simulink library "libMatUdp"  (R2015a)
settings: Solver=ode45  StartTime=0.0  StopTime=10.0  RelTol=1e-3
undefined symbols (not defined in the file): BusSerialize, gcbh, mxpcrtudprx
libraries: xpcnetworkbufferlib x5, xpciplib x4
settings Model: Creator=djoshea  LastModifiedBy=djoshea

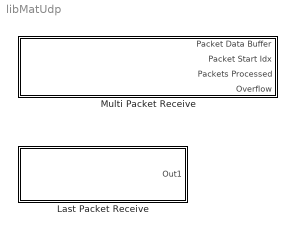
== system libMatUdp ==
  "Last Packet Receive " : Subsystem  InitFcn=mxpcrtudprx(1, get_param(gcbh, 'ID'));  mask(rtudpreceive){maskID=1, sourceIP='0.0.0.0', Receive2=25000, Receive3=1500, Receive4=-1, udpID=0, ID=1}
      mask prompts: maskID "Device ID"; sourceIP "Source IP Address:"; Receive2 "Local (destination) port:"; Receive3 "Output port width:"; Receive4 "Sample time:"; udpID "Internal UDP ID:"; ID "Device ID:"
      mask help:
      | Receive data over UDP network.
      |
      | This block receives data on the specified local (destination) port. To receive all data sent to this port, set 'Source IP Address' to 0.0.0.0. To receive data sent to this port from a specific remote source, enter that IP address.
      mask init:
      | set(gcbh, 'ID', num2str(maskID));
      | set(gcbh, 'Receive1', sourceIP);
      mask TypeOptions Receive2: Receive2
      mask TypeOptions Receive3: Receive3
      mask TypeOptions Receive4: Receive4
      mask TypeOptions udpID: udpID
      mask TypeOptions ID: ID
      mask Display:
      | try
      |     disp(sprintf('UDP Receive\nDevice ID: %d\n%s to port %d', maskID, sourceIP, Receive2));
      | catch
      |     disp('UDP Receive');
      | end
      | port_label('output', 1, 'Data');
  "Multi Packet Receive " : Subsystem  InitFcn=mxpcrtudprx(1, get_param(gcbh, 'ID'));  mask(rtudpreceive){ID=1, sourceIP=0.0.0.0, recvPort=25000, PacketDataBufferMaxSize=15000, PacketChainSize=20, PacketBufferSize=0, Receive4=0.001, udpID=0}
      mask prompts: ID "Device ID:"; sourceIP "Source IP Address:"; recvPort "Local (destination) port:"; PacketDataBufferMaxSize "Packet Data Buffer Max Size:"; PacketChainSize "Packet Chain Size"; PacketBufferSize "Packet Buffer Size"; Receive4 "Sample time:"; udpID "Internal UDP ID:"
      mask help:
      | Receive data over UDP network on a dedicated network interface.
      |
      | This block receives data on the specified local (destination) port. To receive all data sent to this port, set 'Source IP Address' to 0.0.0.0. To receive data sent to this port from a specific remote source, enter the IP address of that source.
      mask init:
      | udpID = ID -1;
      mask Help: eval('xpcdoc(''RT_UDP_RECEIVE'')');
      mask TypeOptions ID: 1 | 2 | 3 | 4 | 5 | 6 | 7 | 8
      mask Display:
      | try
      |     disp(sprintf('Multi-UDP Receive\nDevice Id: %d\n%s to port %d', ...
      |         ID, BusSerialize.ipStringFromAddress(sourceIP), recvPort));
      | catch
      |     disp('Multi-UDP Receive');
      | end
      | port_label('output', 1, 'Data');
      | port_label('output', 2, 'Start Idx');
      | port_label('output', 3, 'Packet Count');
      | port_label('output', 4, 'Overflow');

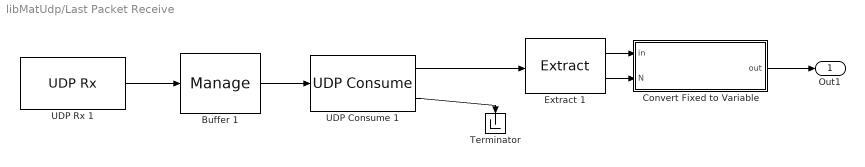
== system libMatUdp/Last Packet Receive  ==
  Buffer 1 : xpcnetworkbufferlib/Manage   ChainSize=-1  BufferSize=0  Threshold=0
  Convert Fixed to Variable : MATLAB Function  TreatAsAtomicUnit=on  mask(Converts Variable-size to fixed-size array){bufferSize=1500}
      mask prompts: bufferSize "Buffer Size"
      mask help: Specify maximum input size.
  Extract 1 : xpcnetworkbufferlib/Extract   PacketSize=Receive3
  Terminator : Terminator
  UDP Consume 1 : xpciplib/UDP Consume   Group=udpID  VectorSize=0  SampleTime=Receive4
  UDP Rx 1 : xpciplib/UDP Rx   Priority=5  Group=udpID  sip=Any  SourceAddress=Receive1  lup=Specify  LocalPort=Receive2  SampleTime=Receive4
  Out1 : Outport  OutDataTypeStr=uint8
  wires:
  Extract 1/1 -> Convert Fixed to Variable/1(in)
  Buffer 1/1 -> UDP Consume 1/1
  UDP Rx 1/1 -> Buffer 1/1
  UDP Consume 1/1 -> Extract 1/1
  UDP Consume 1/2 -> Terminator/1
  Extract 1/2 -> Convert Fixed to Variable/2(N)
  Convert Fixed to Variable/1(out) -> Out1/1

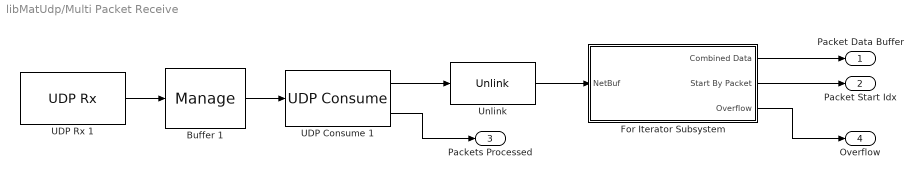
== system libMatUdp/Multi Packet Receive  ==
  Buffer 1 : xpcnetworkbufferlib/Manage   ChainSize=PacketChainSize  BufferSize=PacketBufferSize  Threshold=0
  For Iterator Subsystem : Subsystem  TreatAsAtomicUnit=on
  UDP Consume 1 : xpciplib/UDP Consume   Group=udpID  VectorSize=0  SampleTime=Receive4
  UDP Rx 1 : xpciplib/UDP Rx   Priority=5  Group=udpID  sip=Any  SourceAddress=BusSerialize.ipAddressFromString(sourceIP)  lup=Specify  LocalPort=recvPort  SampleTime=Receive4
  "Unlink " : xpcnetworkbufferlib/Unlink   VectorLength=-1
  Packet Data Buffer : Outport
  Packet Start Idx : Outport  Port=2
  Packets Processed : Outport  Port=3
  Overflow : Outport  Port=4
  wires:
  For Iterator Subsystem/3(Overflow) -> Overflow/1
  For Iterator Subsystem/2(Start By Packet) -> Packet Start Idx/1
  For Iterator Subsystem/1(Combined Data) -> Packet Data Buffer/1
  "Unlink "/1 -> For Iterator Subsystem/1(NetBuf)
  Buffer 1/1 -> UDP Consume 1/1
  UDP Rx 1/1 -> Buffer 1/1
  UDP Consume 1/1 -> "Unlink "/1
  UDP Consume 1/2 -> Packets Processed/1

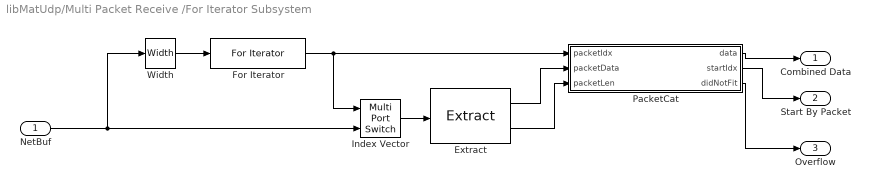
== system libMatUdp/Multi Packet Receive /For Iterator Subsystem ==
  NetBuf : Inport
  "Extract " : xpcnetworkbufferlib/Extract   PacketSize=-1
  For Iterator : ForIterator  ResetStates=reset  IterationSource=external
  Index Vector : MultiPortSwitch  DataPortOrder=Zero-based contiguous  Inputs=1  zeroidx=on
  PacketCat : MATLAB Function  TreatAsAtomicUnit=on
  Width : Width
  Combined Data : Outport
  Start By Packet : Outport  Port=2
  Overflow : Outport  Port=3  OutDataTypeStr=uint8
  wires:
  PacketCat/3(didNotFit) -> Overflow/1
  PacketCat/2(startIdx) -> Start By Packet/1
  PacketCat/1(data) -> Combined Data/1
  "Extract "/2 -> PacketCat/3(packetLen)
  "Extract "/1 -> PacketCat/2(packetData)
  Index Vector/1 -> "Extract "/1
  For Iterator/1 -> PacketCat/1(packetIdx), Index Vector/1
  Width/1 -> For Iterator/1
  NetBuf/1 -> Width/1, Index Vector/2

== matlab function libMatUdp/Multi Packet Receive /For Iterator Subsystem/PacketCat ==
  data: packetIdx input; data output uint8 size=PacketDataBufferMaxSize; packetData input uint8; packetLen input size=1; startIdx output size=PacketChainSize; PacketDataBufferMaxSize parameter size=1; PacketChainSize parameter size=1; didNotFit output uint8 size=1
function [data, startIdx, didNotFit] = packetCat(packetIdx, packetData, packetLen, PacketDataBufferMaxSize, PacketChainSize)
%#codegen

persistent pData;
persistent pDataLen;
persistent pStartIdx;
persistent pStartIdxLen;
persistent pDidNotFit;

if packetIdx == 1 || isempty(pData) || isempty(pDataLen) || isempty(pStartIdx) || isempty(pStartIdxLen) || isempty(pDidNotFit)
    pData = coder.nullcopy(zeros(PacketDataBufferMaxSize, 1, 'uint8'));
    pDataLen = uint32(0);
    pStartIdx = coder.nullcopy(zeros(PacketChainSize, 1, 'uint32'));
    pStartIdxLen = uint16(0);
    pDidNotFit = uint8(0);
end

% check whether there is room for this packet
canFitBytes = numel(pData) - pDataLen >= packetLen;
canFitPacket = numel(pStartIdx) - pStartIdxLen > 0;
if canFitBytes && canFitPacket
    % log the start position of this packet
    packetNum = pStartIdxLen + uint16(1);
    pStartIdx(packetNum) = pDataLen + uint32(1);
    pStartIdxLen = pStartIdxLen + 1;
    
    assert(packetLen <= PacketDataBufferMaxSize);
    
    % and copy this packet into the buffer
    dataIdx = pDataLen + uint32(1:packetLen);
    pData(dataIdx) = packetData(uint32(1:packetLen));
    pDataLen = pDataLen + packetLen;
else
    pDidNotFit = uint8(1);
end

data = pData(1:pDataLen);
startIdx = pStartIdx(1:pStartIdxLen);
didNotFit = pDidNotFit;

== matlab function libMatUdp/Last Packet Receive /Convert Fixed to Variable ==
  data: in input; out output size=bufferSize; N input size=1; bufferSize parameter size=1
function out = fixedToVariable(in, N, bufferSize)
%#codegen

if N == 0
    out = zeros(0, 1, class(in)); %#ok<ZEROLIKE>
elseif N > bufferSize
    out = in;
else
    out = in(1:N);
end
